simulink model "PID_emulation_be_ff"  (R2022b)
settings: Solver=ode45  StartTime=0.0  StopTime=5  RelTol=1e-3
values from neighbouring files (symbols this model uses):
  degs2rpm = 0.166666666667    [parameters.mat]
  der =     [parameters.mat]
  drv =     [parameters.mat]
  gbox =     [parameters.mat]
  mot =     [parameters.mat]
  real =     [parameters.mat]
  rpm2degs = 6    [parameters.mat]
  rpm2rads = 0.10471975512    [parameters.mat]
  sens =     [parameters.mat]
  simul =     [parameters.mat]
  Ts = 0.001    [parameters.mat]
undefined symbols (not defined in the file or in its folder): DiscIntNeverNeededParam, pidz, T
libraries: simulink x1
settings Model: Creator=emanuelevitetta  LastModifiedBy=michael

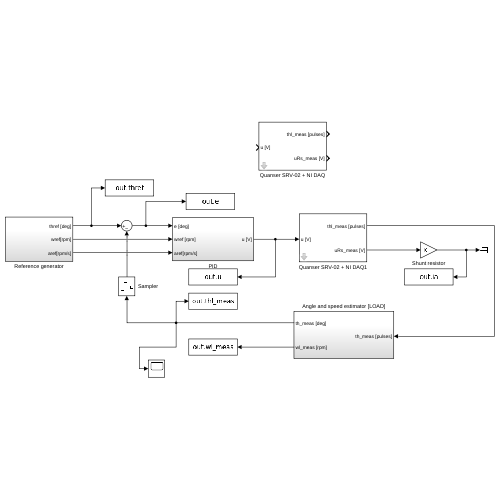
[thumbnail: Simulink's stored preview of the top-level diagram]
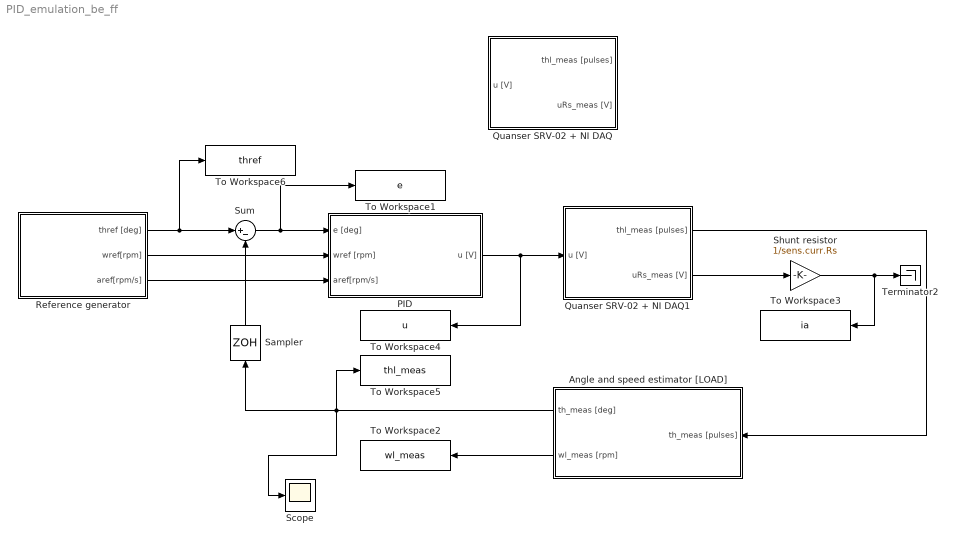
== system PID_emulation_be_ff ==
  Angle and speed estimator [LOAD] : Subsystem
  PID : Subsystem
  Quanser SRV-02 + NI DAQ : Subsystem  mask(Quanser SRV-02 (with inertial load) + NI DAQ){Ts=0.001, fricType=Coulomb + viscous}
      mask prompts: Ts "NI DAQ Sample Time:"; fricType "Friction model"
      mask help: Quanser SRV-02 (with inertial load) + NI DAQ model.
      mask init:
      | %%  Sensors data
      | 
      | %   shunt resistor
      | sens.curr.Rs = 0.5;                         %   resistance [Ohm]   
      | sens.curr.uRs_std = 0.01;                   %   voltage noise standard dev [V]                           
      | sens.curr.uRs_var = sens.curr.uRs_std^2;	%   voltage noise variance [V^2]
      | 
      | %   Hewlett-Packard HEDS-5540#A06 optical encoder
      | sens.enc.ppr = 500*4;                       %   pulses per rotation
      | sens.enc.pulse2deg = 360/sens.enc.ppr;      %   [pulses] -> [deg]
      | sens.enc.pulse2rad = 2*pi/sens.enc.ppr;     %   [pulses] -> [rad]
      | sens.enc.deg2pulse = sens.enc.ppr/360;      %   [deg] -> [pulses]
      | sens.enc.rad2pulse = sens.enc.ppr/2/pi;     %   [rad] -> [pulses]
      | 
      | 
      | %%  Data acquisition board (daq) data
      | 
      | %   NI PCI-6221 DAC data
      | daq.dac.bits = 16;                                  %   resolution (bits)
      | daq.dac.fs   = 10;                                  %   full scale 
      | daq.dac.q    = 2*daq.dac.fs/(2^daq.dac.bits-1);     %	quantization
      | 
      | %   NI PCI-6221 ADC data
      | daq.adc.bits = 16;                                  %   resolution (bits)
      | daq.adc.fs   = 10;                                  %   full scale (as set in SLDRT Analog Input block)
      | daq.adc.q    = 2*daq.adc.fs/(2^daq.adc.bits-1);     %   quantization
      mask Help:
      | Riccardo Antonello (antonello@dei.unipd.it)
      | 
      | April 24, 2020
      | 
      | Dept. of Information Engineering, University of Padova
      mask TypeOptions fricType: Coulomb + viscous | Karnopp
  Quanser SRV-02 + NI DAQ1 : Subsystem  mask(Quanser SRV-02 (with inertial load) + NI DAQ){Ts=0.001, fricType=Coulomb + viscous}
      mask prompts: Ts "NI DAQ Sample Time:"; fricType "Friction model"
      mask help: Quanser SRV-02 (with inertial load) + NI DAQ model.
      mask init: same as PID_emulation_be_ff/Quanser SRV-02 + NI DAQ
      mask Help:
      | Riccardo Antonello (antonello@dei.unipd.it)
      | 
      | April 24, 2020
      | 
      | Dept. of Information Engineering, University of Padova
      mask TypeOptions fricType: Coulomb + viscous | Karnopp
  Reference generator : Subsystem
  Sampler : ZeroOrderHold  SampleTime=T(simul.Ts_selector)
  Scope : Scope
  Shunt resistor : Gain  Gain=1/sens.curr.Rs
  Sum : Sum  Inputs=|+-
  Terminator2 : Terminator
  To Workspace1 : ToWorkspace  VariableName=e  SaveFormat=Structure With Time  SampleTime=Ts
  To Workspace2 : ToWorkspace  VariableName=wl_meas  SaveFormat=Structure With Time  SampleTime=Ts
  To Workspace3 : ToWorkspace  VariableName=ia  SaveFormat=Structure With Time  SampleTime=Ts
  To Workspace4 : ToWorkspace  VariableName=u  SaveFormat=Structure With Time  SampleTime=Ts
  To Workspace5 : ToWorkspace  VariableName=thl_meas  SaveFormat=Structure With Time  SampleTime=Ts
  To Workspace6 : ToWorkspace  VariableName=thref  SaveFormat=Structure With Time  SampleTime=Ts
  wires:
  PID/1(u [V]) -> Quanser SRV-02 + NI DAQ1/1(u [V]), To Workspace4/1
  Sum/1 -> To Workspace1/1, PID/1(e [deg])
  Shunt resistor/1 -> To Workspace3/1, Terminator2/1
  Reference generator/1(thref [deg]) -> To Workspace6/1, Sum/1
  Quanser SRV-02 + NI DAQ1/1(thl_meas [pulses]) -> Angle and speed estimator [LOAD]/1(th_meas [pulses])
  Angle and speed estimator [LOAD]/1(th_meas [deg]) -> Scope/1, Sampler/1, To Workspace5/1
  Angle and speed estimator [LOAD]/2(wl_meas [rpm]) -> To Workspace2/1
  Reference generator/2(wref[rpm]) -> PID/2(wref [rpm])
  Reference generator/3(aref[rpm/s]) -> PID/3(aref[rpm/s])
  Sampler/1 -> Sum/2
  Quanser SRV-02 + NI DAQ1/2(uRs_meas [V]) -> Shunt resistor/1

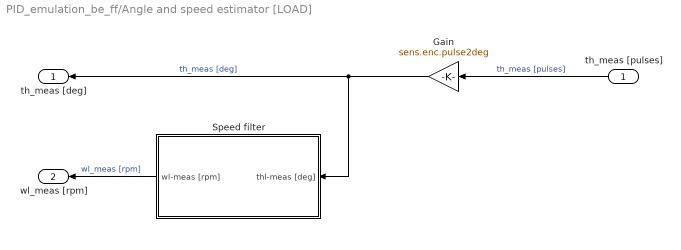
== system PID_emulation_be_ff/Angle and speed estimator [LOAD] ==
  th_meas [pulses] : Inport
  Gain : Gain  Gain=sens.enc.pulse2deg
  Speed filter : Subsystem
  th_meas [deg] : Outport
  wl_meas [rpm] : Outport  Port=2
  wires:
  Speed filter/1(wl-meas [rpm]) -> wl_meas [rpm]/1  "wl_meas [rpm]"
  th_meas [pulses]/1 -> Gain/1  "th_meas [pulses]"
  Gain/1 -> Speed filter/1(thl-meas [deg]), th_meas [deg]/1  "th_meas [deg]"

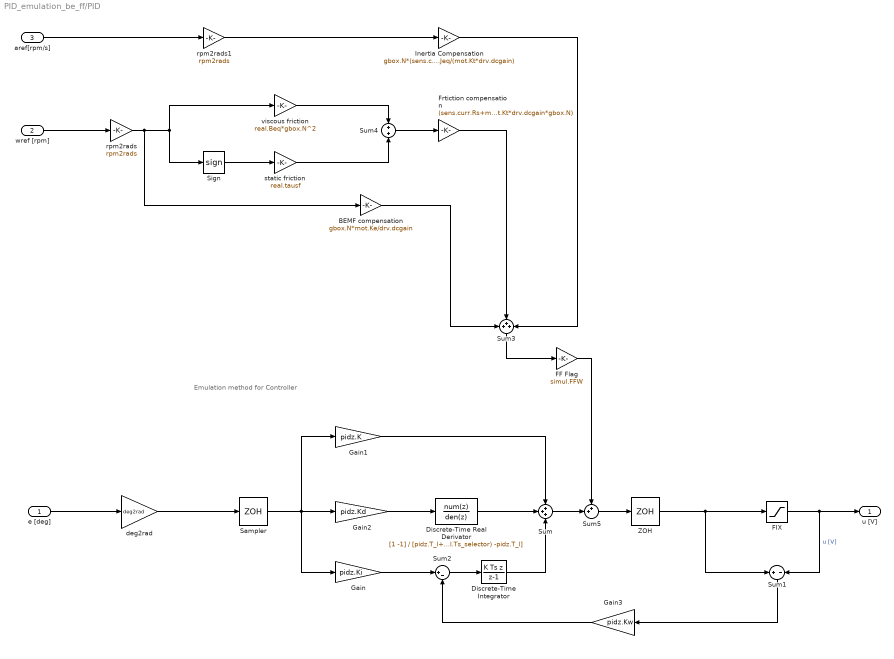
== system PID_emulation_be_ff/PID ==
  note: Emulation method for Controller
  e [deg] : Inport
  wref [rpm] : Inport  Port=2
  aref[rpm/s] : Inport  Port=3
  BEMF compensation : Gain  Gain=gbox.N*mot.Ke/drv.dcgain
  Discrete-Time Integrator : DiscreteIntegrator  IntegratorMethod=Integration: Backward Euler  SampleTime=T(simul.Ts_selector)  ICPrevOutput=DiscIntNeverNeededParam  ICPrevScaledInput=DiscIntNeverNeededParam
  "Discrete-Time Real Derivator " : DiscreteTransferFcn  Numerator=[1 -1]  Denominator=[pidz.T_l+T(simul.Ts_selector) -pidz.T_l]  SampleTime=T(simul.Ts_selector)
  FF Flag : Gain  Gain=simul.FFW
  "FIX " : Saturate  UpperLimit=10  LowerLimit=-10
  Frtiction compensation : Gain  Gain=(sens.curr.Rs+mot.R)/(mot.Kt*drv.dcgain*gbox.N)
  Gain : Gain  Gain=pidz.Ki
  Gain1 : Gain  Gain=pidz.K
  Gain2 : Gain  Gain=pidz.Kd
  Gain3 : Gain  Gain=pidz.Kw
  Inertia Compensation : Gain  Gain=gbox.N*(sens.curr.Rs+mot.R)*real.Jeq/(mot.Kt*drv.dcgain)
  Sampler : ZeroOrderHold  SampleTime=T(simul.Ts_selector)
  Sign : Signum
  Sum : Sum  Inputs=+++
  Sum1 : Sum  Inputs=+|-
  Sum2 : Sum  Inputs=|+-
  Sum3 : Sum  Inputs=+++
  Sum4 : Sum
  Sum5 : Sum  Inputs=++|
  ZOH : ZeroOrderHold  SampleTime=T(simul.Ts_selector)
  deg2rad : Gain  Gain=deg2rad
  rpm2rads : Gain  Gain=rpm2rads
  rpm2rads1 : Gain  Gain=rpm2rads
  static friction : Gain  Gain=real.tausf
  viscous friction : Gain  Gain=real.Beq*gbox.N^2
  u [V] : Outport
  wires:
  e [deg]/1 -> deg2rad/1
  "FIX "/1 -> Sum1/2, u [V]/1  "u [V]"
  deg2rad/1 -> Sampler/1
  ZOH/1 -> Sum1/1, "FIX "/1
  Gain2/1 -> "Discrete-Time Real Derivator "/1
  Sampler/1 -> Gain2/1, Gain1/1, Gain/1
  Gain1/1 -> Sum/1
  "Discrete-Time Real Derivator "/1 -> Sum/2
  Discrete-Time Integrator/1 -> Sum/3
  Gain/1 -> Sum2/1
  Sum2/1 -> Discrete-Time Integrator/1
  Sum1/1 -> Gain3/1
  Gain3/1 -> Sum2/2
  static friction/1 -> Sum4/2
  wref [rpm]/1 -> rpm2rads/1
  Sign/1 -> static friction/1
  rpm2rads1/1 -> Inertia Compensation/1
  Inertia Compensation/1 -> Sum3/3
  BEMF compensation/1 -> Sum3/1
  rpm2rads/1 -> BEMF compensation/1, Sign/1, viscous friction/1
  aref[rpm/s]/1 -> rpm2rads1/1
  viscous friction/1 -> Sum4/1
  Frtiction compensation/1 -> Sum3/2
  Sum4/1 -> Frtiction compensation/1
  Sum3/1 -> FF Flag/1
  Sum/1 -> Sum5/2
  FF Flag/1 -> Sum5/1
  Sum5/1 -> ZOH/1

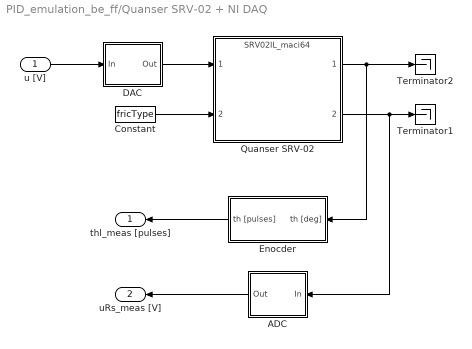
== system PID_emulation_be_ff/Quanser SRV-02 + NI DAQ ==
  u [V] : Inport
  ADC : Subsystem
  Constant : Constant  Value=fricType
  DAC : Subsystem
  Enocder : Subsystem
  Quanser SRV-02 : ModelReference  ModelNameDialog=SRV02IL_maci64.slxp  ModelReferenceVersion=1.44  CopyOfModelProtected=on
  Terminator1 : Terminator
  Terminator2 : Terminator
  thl_meas [pulses] : Outport
  uRs_meas [V] : Outport  Port=2
  wires:
  Enocder/1(th [pulses]) -> thl_meas [pulses]/1
  ADC/1(Out) -> uRs_meas [V]/1
  DAC/1(Out) -> Quanser SRV-02/1
  Quanser SRV-02/2 -> ADC/1(In), Terminator1/1
  u [V]/1 -> DAC/1(In)
  Quanser SRV-02/1 -> Enocder/1(th [deg]), Terminator2/1
  Constant/1 -> Quanser SRV-02/2

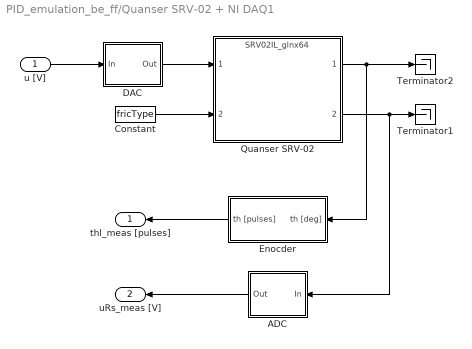
== system PID_emulation_be_ff/Quanser SRV-02 + NI DAQ1 ==
  u [V] : Inport
  ADC : Subsystem
  Constant : Constant  Value=fricType
  DAC : Subsystem
  Enocder : Subsystem
  Quanser SRV-02 : ModelReference  ModelNameDialog=SRV02IL_glnx64.slxp  ModelReferenceVersion=1.45  CopyOfModelProtected=on
  Terminator1 : Terminator
  Terminator2 : Terminator
  thl_meas [pulses] : Outport
  uRs_meas [V] : Outport  Port=2
  wires:
  Enocder/1(th [pulses]) -> thl_meas [pulses]/1
  ADC/1(Out) -> uRs_meas [V]/1
  DAC/1(Out) -> Quanser SRV-02/1
  Quanser SRV-02/2 -> ADC/1(In), Terminator1/1
  u [V]/1 -> DAC/1(In)
  Quanser SRV-02/1 -> Enocder/1(th [deg]), Terminator2/1
  Constant/1 -> Quanser SRV-02/2

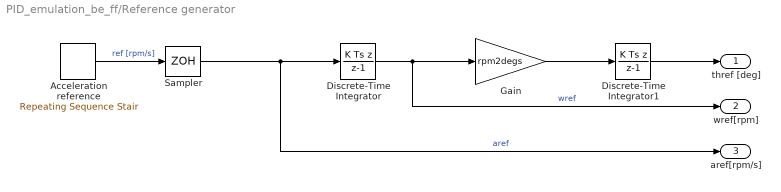
== system PID_emulation_be_ff/Reference generator ==
  Acceleration reference : simulink/Sources/Repeating Sequence Stair  OutValues=[900 0 -900 -900 0 900].'  tsamp=0.5  OutMin=[]  OutMax=[]  OutDataTypeStr=double  OutputDataTypeScalingMode=double  OutDataType=fixdt(0,8)  ConRadixGroup=Best Precision: Vector-wise  OutScaling=2^-12
  Discrete-Time Integrator : DiscreteIntegrator  IntegratorMethod=Integration: Backward Euler  SampleTime=-1  ICPrevOutput=DiscIntNeverNeededParam  ICPrevScaledInput=DiscIntNeverNeededParam
  Discrete-Time Integrator1 : DiscreteIntegrator  IntegratorMethod=Integration: Backward Euler  SampleTime=-1  ICPrevOutput=DiscIntNeverNeededParam  ICPrevScaledInput=DiscIntNeverNeededParam
  Gain : Gain  Gain=rpm2degs
  Sampler : ZeroOrderHold  SampleTime=T(simul.Ts_selector)
  thref [deg] : Outport
  wref[rpm] : Outport  Port=2
  aref[rpm/s] : Outport  Port=3
  wires:
  Acceleration reference/1 -> Sampler/1  "ref [rpm/s]"
  Sampler/1 -> aref[rpm/s]/1, Discrete-Time Integrator/1  "aref"
  Discrete-Time Integrator/1 -> wref[rpm]/1, Gain/1  "wref"
  Discrete-Time Integrator1/1 -> thref [deg]/1
  Gain/1 -> Discrete-Time Integrator1/1

== system PID_emulation_be_ff/Angle and speed estimator [LOAD]/Speed filter ==
  thl-meas [deg] : Inport
  Real Derivative : TransferFcn  Numerator=[der.wc^2 0]  Denominator=[1 2*der.d*der.wc der.wc^2]
  degs2rpm : Gain  Gain=degs2rpm
  wl-meas [rpm] : Outport
  wires:
  thl-meas [deg]/1 -> Real Derivative/1
  degs2rpm/1 -> wl-meas [rpm]/1  "wl-meas"
  Real Derivative/1 -> degs2rpm/1

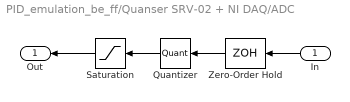
== system PID_emulation_be_ff/Quanser SRV-02 + NI DAQ/ADC ==
  In : Inport
  Quantizer : Quantizer  QuantizationInterval=daq.adc.q
  Saturation : Saturate  UpperLimit=daq.adc.fs  LowerLimit=-daq.adc.fs
  Zero-Order Hold : ZeroOrderHold  SampleTime=Ts
  Out : Outport
  wires:
  Saturation/1 -> Out/1
  In/1 -> Zero-Order Hold/1
  Quantizer/1 -> Saturation/1
  Zero-Order Hold/1 -> Quantizer/1

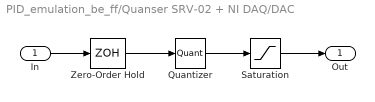
== system PID_emulation_be_ff/Quanser SRV-02 + NI DAQ/DAC ==
  In : Inport
  Quantizer : Quantizer  QuantizationInterval=daq.dac.q
  Saturation : Saturate  UpperLimit=daq.dac.fs  LowerLimit=-daq.dac.fs
  Zero-Order Hold : ZeroOrderHold  SampleTime=Ts
  Out : Outport
  wires:
  Quantizer/1 -> Saturation/1
  In/1 -> Zero-Order Hold/1
  Zero-Order Hold/1 -> Quantizer/1
  Saturation/1 -> Out/1

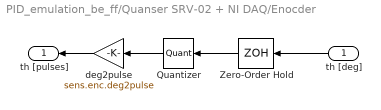
== system PID_emulation_be_ff/Quanser SRV-02 + NI DAQ/Enocder ==
  th [deg] : Inport
  Quantizer : Quantizer  QuantizationInterval=sens.enc.pulse2deg
  Zero-Order Hold : ZeroOrderHold  SampleTime=Ts
  deg2pulse : Gain  Gain=sens.enc.deg2pulse
  th [pulses] : Outport
  wires:
  Quantizer/1 -> deg2pulse/1
  th [deg]/1 -> Zero-Order Hold/1
  Zero-Order Hold/1 -> Quantizer/1
  deg2pulse/1 -> th [pulses]/1

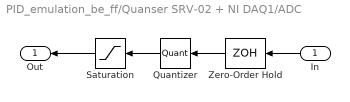
== system PID_emulation_be_ff/Quanser SRV-02 + NI DAQ1/ADC ==
  In : Inport
  Quantizer : Quantizer  QuantizationInterval=daq.adc.q
  Saturation : Saturate  UpperLimit=daq.adc.fs  LowerLimit=-daq.adc.fs
  Zero-Order Hold : ZeroOrderHold  SampleTime=Ts
  Out : Outport
  wires:
  Saturation/1 -> Out/1
  In/1 -> Zero-Order Hold/1
  Quantizer/1 -> Saturation/1
  Zero-Order Hold/1 -> Quantizer/1

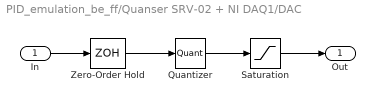
== system PID_emulation_be_ff/Quanser SRV-02 + NI DAQ1/DAC ==
  In : Inport
  Quantizer : Quantizer  QuantizationInterval=daq.dac.q
  Saturation : Saturate  UpperLimit=daq.dac.fs  LowerLimit=-daq.dac.fs
  Zero-Order Hold : ZeroOrderHold  SampleTime=Ts
  Out : Outport
  wires:
  Quantizer/1 -> Saturation/1
  In/1 -> Zero-Order Hold/1
  Zero-Order Hold/1 -> Quantizer/1
  Saturation/1 -> Out/1

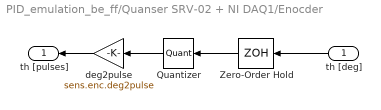
== system PID_emulation_be_ff/Quanser SRV-02 + NI DAQ1/Enocder ==
  th [deg] : Inport
  Quantizer : Quantizer  QuantizationInterval=sens.enc.pulse2deg
  Zero-Order Hold : ZeroOrderHold  SampleTime=Ts
  deg2pulse : Gain  Gain=sens.enc.deg2pulse
  th [pulses] : Outport
  wires:
  Quantizer/1 -> deg2pulse/1
  th [deg]/1 -> Zero-Order Hold/1
  Zero-Order Hold/1 -> Quantizer/1
  deg2pulse/1 -> th [pulses]/1
